simulink model "ModbusReceive"  (R2022a)
settings: Solver=FixedStepDiscrete  StartTime=0.0  StopTime=inf  FixedStep=0.2  RelTol=1e-3
undefined symbols (not defined in the file): now
settings Model: Creator=Sajid Ali  LastModifiedBy=Sajid Ali

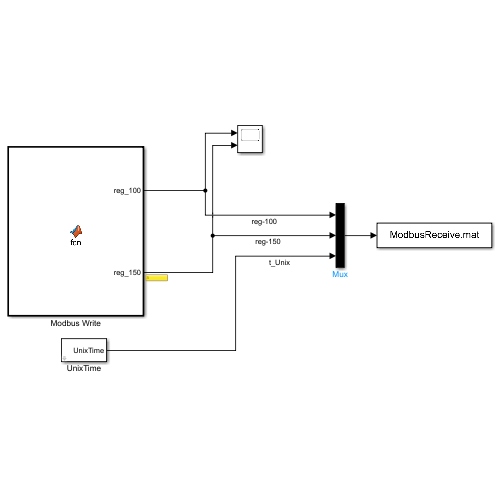
[thumbnail: Simulink's stored preview of the top-level diagram]
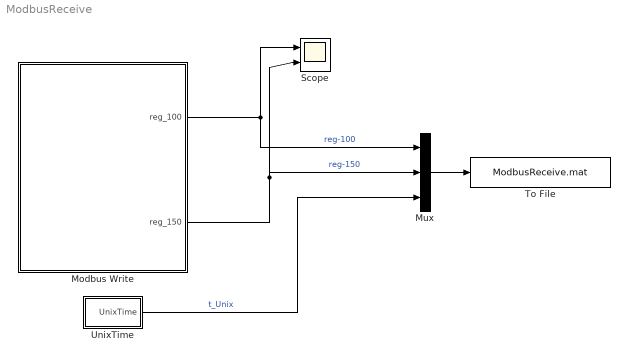
== system ModbusReceive ==
  Modbus Write : MATLAB Function  TreatAsAtomicUnit=on  SystemSampleTime=1
  Mux : Mux  Inputs=3
  Scope : Scope  NumInputPorts=2
  To File : ToFile  Filename=ModbusReceive.mat  SaveFormat=Timeseries
  UnixTime : Subsystem
      mask DialogControl DescGroupVar Prompt: Description
      mask DialogControl DescTextVar Prompt: This system provides the unix time stamp.  Unix time is a system for describing a point in time. It is the number of seconds that have elapsed since the Unix epoch, excluding leap seconds. The Unix epoch is 00:00:00 UTC on 1 January 1970. Madeby: Sajid Ali : sajidali75092@gmail.com
      mask DialogControl ParameterGroupVar Prompt: No Parameters needed
  wires:
  UnixTime/1(UnixTime) -> Mux/3  "t_Unix"
  Modbus Write/2(reg_150) -> Scope/2, Mux/2  "reg-150"
  Mux/1 -> To File/1
  Modbus Write/1(reg_100) -> Mux/1, Scope/1  "reg-100"

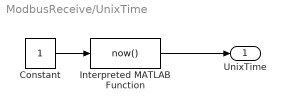
== system ModbusReceive/UnixTime ==
  Constant : Constant
  Interpreted MATLAB Function : MATLABFcn  MATLABFcn=now()
  UnixTime : Outport
  wires:
  Interpreted MATLAB Function/1 -> UnixTime/1
  Constant/1 -> Interpreted MATLAB Function/1

== matlab function ModbusReceive/Modbus Write ==
  settings: updateMethod=DISCRETE  sampleTime=1
  data: reg_100 output; reg_150 output
function [reg_100,reg_150]=fcn()

persistent m;



if isempty(m)
    m = modbus('tcpip','192.168.100.173','Timeout',3,'NumRetries',10);
end

%Syntax
% read(var, 'holdingregs', reg_address, 1, serverId, 'int16');

a=read(m, 'holdingregs', 101, 1, 1, 'int16');
b=read(m, 'holdingregs', 151, 1, 1, 'int16');
reg_100=a(1);
reg_150=b(1);
